simulink model "City_Env_2Car_CS2020"  (Simulink 9.3)
settings: Solver=ode45  StartTime=0  StopTime=20  RelTol=1e-3  EnableMultiTasking=on
libraries: Solver_SF x2
settings Model: Creator=dhall  LastModifiedBy=msayers  ExtModeTrigMode=oneshot  ExtModeArmWhenConnect=off
settings DataIOCC: SignalLoggingName=sigsOut
settings OptimizationCC: BooleanDataType=off  LocalBlockOutputs=off  InitFltsAndDblsToZero=on
settings DebuggingCC: SaveWithParameterizedLinksMsg=none  SignalResolutionControl=TryResolveAllWithWarning  MultiTaskDSMMsg=warning  MultiTaskCondExecSysMsg=none  StateNameClashWarn=warning
settings HardwareCC: TargetUnknown=on
settings GRTTargetCC: TargetFcnLib=ansi_tfl_tmw.mat  CompOptLevelCompliant=off  GeneratePreprocessorConditionals=Disable all

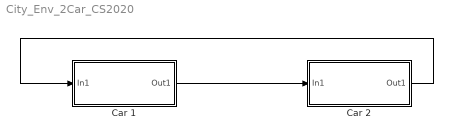
== system City_Env_2Car_CS2020 ==
  Car 1 : Subsystem
  Car 2 : Subsystem
  wires:
  Car 1/1(Out1) -> Car 2/1(In1)
  Car 2/1(Out1) -> Car 1/1(In1)

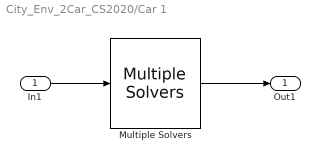
== system City_Env_2Car_CS2020/Car 1 ==
  In1 : Inport
  Multiple Solvers : Solver_SF/Multiple Solvers  Priority=1  iVehicle=1  SIMFILE=D:\product_dev\trunk\Image\CarSim\Core\CarSim_Data\simfile1.sim  Run_RTs=off  vs_state_ind=Run  StopMode_ind=Vehicle Model  vs_scx=on
  Out1 : Outport
  wires:
  In1/1 -> Multiple Solvers/1
  Multiple Solvers/1 -> Out1/1

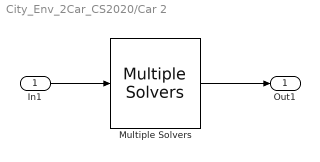
== system City_Env_2Car_CS2020/Car 2 ==
  In1 : Inport
  Multiple Solvers : Solver_SF/Multiple Solvers  Priority=1  iVehicle=2  SIMFILE=D:\product_dev\trunk\Image\CarSim\Core\CarSim_Data\simfile2.sim  Run_RTs=off  vs_state_ind=Run  StopMode_ind=Vehicle Model  vs_scx=on
  Out1 : Outport
  wires:
  In1/1 -> Multiple Solvers/1
  Multiple Solvers/1 -> Out1/1
